simulink model "SimulinkEx1"  (R2024a)
settings: Solver=VariableStepAuto  StartTime=0.0  StopTime=10.0  RelTol=1e-3
values from neighbouring files (symbols this model uses):
  A = [0, 1; -10.5, -11.3]    [Ex1.m]
  Ae = [A, zeros(2,1) ... (first row only)    [Ex1.m]
  B = [0; 0.55]    [Ex1.m]
  Be = [B; 0]    [Ex1.m]
  C = [1, 0]    [Ex1.m]
  Ce = [C, 0]    [Ex1.m]
  K = Kc(1:2)    [Ex1.m]
  Ke = acker(sys_dual.A, sys_dual.B, po')'    [Ex1.m]
  Ki = -Kc(3)    [Ex1.m]
settings Model: Creator=caugu  LastModifiedBy=caugu

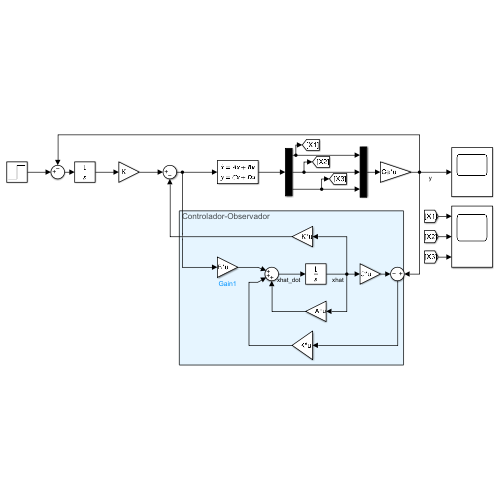
[thumbnail: Simulink's stored preview of the top-level diagram]
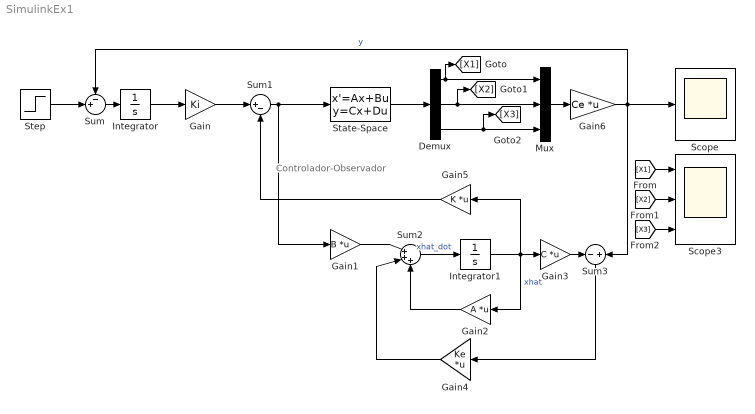
== system SimulinkEx1 ==
  note: Controlador-Observador
  Demux : Demux  Outputs=3
  Gain : Gain  Gain=Ki
  Gain1 : Gain  Gain=B  Multiplication=Matrix(K*u)
  Gain2 : Gain  Gain=A  Multiplication=Matrix(K*u)
  Gain3 : Gain  Gain=C  Multiplication=Matrix(K*u)
  Gain4 : Gain  Gain=Ke  Multiplication=Matrix(K*u)
  Gain5 : Gain  Gain=K  Multiplication=Matrix(K*u)
  Gain6 : Gain  Gain=Ce  Multiplication=Matrix(K*u)
  Integrator : Integrator
  Integrator1 : Integrator
  Mux : Mux  Inputs=3
  Scope : Scope
  Scope3 : Scope  NumInputPorts=3
  State-Space : StateSpace  A=Ae  B=Be  C=eye(3)  D=zeros(3,1)  InitialCondition=0
  Step : Step  Time=0  SampleTime=0
  Sum : Sum  Inputs=-+|
  Sum1 : Sum  Inputs=|+-
  Sum2 : Sum  Inputs=|+++
  Sum3 : Sum  Inputs=-+
  wires:
  Gain4/1 -> Sum2/2
  State-Space/1 -> Demux/1
  Sum/1 -> Integrator/1
  Integrator1/1 -> Gain3/1, Gain5/1, Gain2/1  "xhat"
  Gain/1 -> Sum1/1
  Sum3/1 -> Gain4/1
  Gain2/1 -> Sum2/3
  Gain3/1 -> Sum3/1
  Step/1 -> Sum/2
  Demux/3 -> [X3], Mux/3
  Integrator/1 -> Gain/1
  Demux/1 -> [X1], Mux/1
  Gain6/1 -> Sum3/2, Scope/1, Sum/1  "y"
  Mux/1 -> Gain6/1
  Sum1/1 -> State-Space/1, Gain1/1
  Demux/2 -> [X2], Mux/2
  Gain5/1 -> Sum1/2
  Sum2/1 -> Integrator1/1  "xhat_dot"
  Gain1/1 -> Sum2/1
  [X1] -> Scope3/1
  [X2] -> Scope3/2
  [X3] -> Scope3/3
